simulink model "testNovint_PID"  (R2014b)
settings: Solver=FixedStepDiscrete  StartTime=0.0  StopTime=inf  FixedStep=0.001  RelTol=1e-3
libraries: roblocks x1, LibrarySimulinkSAS x1, rtwinlib x1
settings Model: Creator=Usuario  LastModifiedBy=emanuel
settings DataIOCC: SignalLoggingSaveFormat=ModelDataLogs
settings OptimizationCC: ExpressionDepthLimit=2147483647
settings DebuggingCC: UnderspecifiedInitializationDetection=Classic  MergeDetectMultiDrivingBlocksExec=none  FcnCallInpInsideContextMsg=UseLocalSettings  StateNameClashWarn=warning
settings GRTTargetCC: CombineOutputUpdateFcns=off  GRTInterface=on

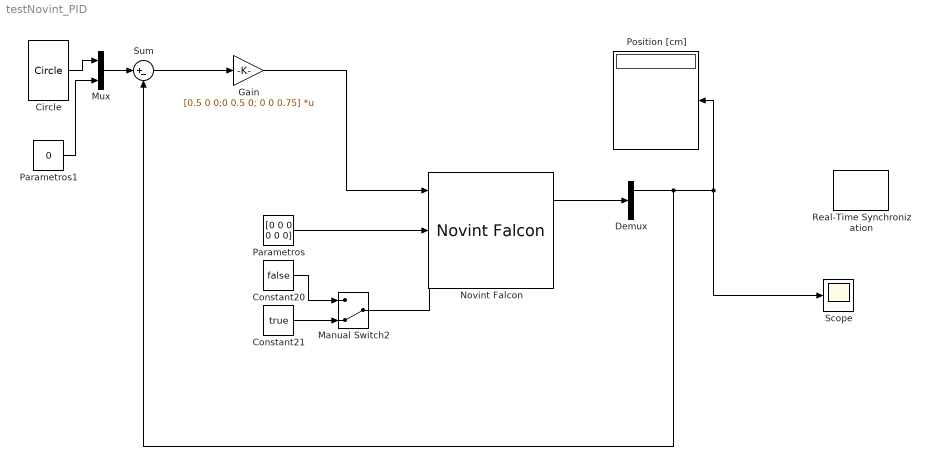
== system testNovint_PID ==
  Circle : roblocks/Trajectory/Circle  radius=2  freq=0.5
  Constant20 : Constant  Value=false
  Constant21 : Constant  Value=true
  Demux : Demux  Outputs=2
  Gain : Gain  Gain=[0.5 0 0;0 0.5 0; 0 0 0.75]  Multiplication=Matrix(K*u) (u vector)
  Manual Switch2 : ManualSwitch  CurrentSetting=0
  Mux : Mux  Inputs=2
  Novint Falcon : LibrarySimulinkSAS/Novint Falcon  dev=1
  Parametros : Constant  Value=[0 0 0 0 0 0]  SampleTime=-1
  Parametros1 : Constant  Value=0  SampleTime=-1
  Position [cm] : Display
  Real-Time Synchronization : rtwinlib/Real-Time Synchronization  SampleTime=0.1  MaxMissedTicks=inf  ShowMissedTicks=off  YieldWhenWaiting=off
  Scope : Scope
      settings: YMax=4
  Sum : Sum  Inputs=|+-
  wires:
  Constant20/1 -> Manual Switch2/1
  Constant21/1 -> Manual Switch2/2
  Manual Switch2/1 -> Novint Falcon/3
  Parametros/1 -> Novint Falcon/2
  Novint Falcon/1 -> Demux/1
  Demux/1 -> Sum/2, Scope/1, Position [cm]/1
  Mux/1 -> Sum/1
  Circle/1 -> Mux/1
  Parametros1/1 -> Mux/2
  Sum/1 -> Gain/1
  Gain/1 -> Novint Falcon/1
